simulink model "Timing"  (R2022a)
settings: Solver=FixedStepAuto  StartTime=0.0  StopTime=0.005  RelTol=1e-3
settings Model: Creator=Mechatronics  LastModifiedBy=Mechatronics

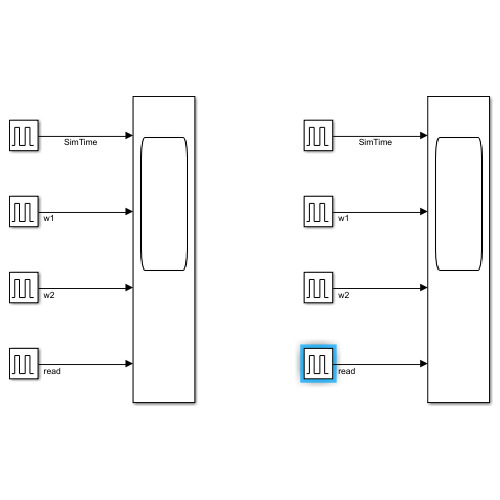
[thumbnail: Simulink's stored preview of the top-level diagram]
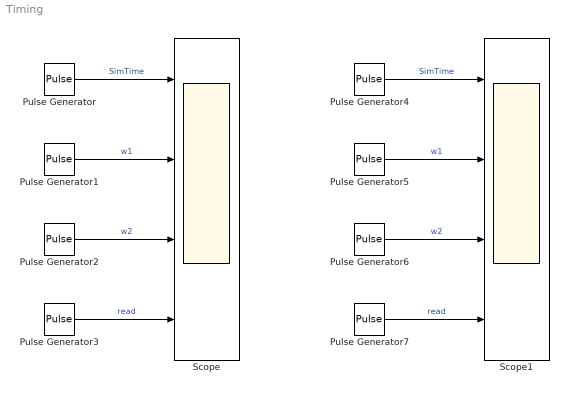
== system Timing ==
  Pulse Generator : DiscretePulseGenerator  PulseType=Time based  Period=1/2000  PulseWidth=50
  Pulse Generator1 : DiscretePulseGenerator  PulseType=Time based  Period=1/500  PulseWidth=50
  Pulse Generator2 : DiscretePulseGenerator  PulseType=Time based  Period=1/500  PulseWidth=50  PhaseDelay=1/(500*2)
  Pulse Generator3 : DiscretePulseGenerator  PulseType=Time based  Period=1/1000  PulseWidth=50  PhaseDelay=1/(4*500)
  Pulse Generator4 : DiscretePulseGenerator  PulseType=Time based  Period=1/(700*4)  PulseWidth=50
  Pulse Generator5 : DiscretePulseGenerator  PulseType=Time based  Period=1/700  PulseWidth=50
  Pulse Generator6 : DiscretePulseGenerator  PulseType=Time based  Period=1/700  PulseWidth=50  PhaseDelay=1/(600*2)
  Pulse Generator7 : DiscretePulseGenerator  PulseType=Time based  Period=1/600  PulseWidth=50  PhaseDelay=1/(4*600)
  Scope : Scope  NumInputPorts=4
  Scope1 : Scope  NumInputPorts=4
  wires:
  Pulse Generator/1 -> Scope/1  "SimTime"
  Pulse Generator1/1 -> Scope/2  "w1"
  Pulse Generator2/1 -> Scope/3  "w2"
  Pulse Generator3/1 -> Scope/4  "read"
  Pulse Generator5/1 -> Scope1/2  "w1"
  Pulse Generator6/1 -> Scope1/3  "w2"
  Pulse Generator7/1 -> Scope1/4  "read"
  Pulse Generator4/1 -> Scope1/1  "SimTime"
